simulink model "Disc"  (R2016b)
settings: Solver=VariableStepAuto  StartTime=0.0  StopTime=inf  RelTol=1e-3
undefined symbols (not defined in the file or in its folder): gray, Horn, Rec, Schunck, SDTV
libraries: visionstatistics x1, visionconversions x1, visiontextngfix x1, dspvision x1, visionanalysis x1
settings Model: Creator=shaurya  LastModifiedBy=Anushri-MacBook

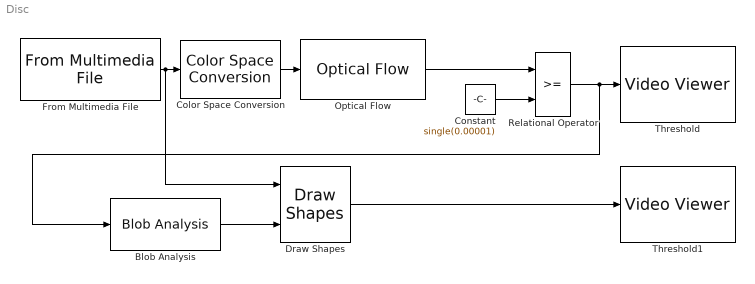
== system Disc ==
  " Threshold" : VideoViewer  colormapValue=gray(256)  FigPos=[617 607 476 443]  trueSizedOnce=on
  " Threshold1" : VideoViewer  colormapValue=gray(256)  FigPos=[140 607 476 443]  trueSizedOnce=on
  Blob Analysis : visionstatistics/Blob Analysis  Tag=vipblks_row_conv  area=off  centroid=off  bBox=on  majorAxis=off  minorAxis=off  angle=off  eccentricity=off  equivDiameterSq=off  extent=off  perimeter=off  maxBlobs=80  warnIfNumBlobsExceeded=on  isCount=off  useMinArea=on  minArea=200  useMaxArea=on  maxArea=400  excludeBorderBlob=on  outDT=double  isOutVarDim=on  isFill=on  fillValues=-1  conn=4  isLabel=off  outputMode=Binary point scaling  outputWordLength=32  outputFracLength=16  firstCoeffMode=Binary point scaling  firstCoeffWordLength=16  firstCoeffFracLength=14  secondCoeffMode=Binary point scaling  secondCoeffWordLength=32  secondCoeffFracLength=16  accumMode=Binary point scaling  accumWordLength=32  accumFracLength=0  prodOutputMode=Binary point scaling  prodOutputWordLength=32  prodOutputFracLength=16  roundingMode=Floor  overflowMode=off
  Color Space Conversion : visionconversions/Color Space  Conversion  conversion=Obsolete  conversionActive=R'G'B' to intensity  wp_str=D65  rec=Rec. 601 (SDTV)  sys=1125/60/2:1  imagePorts=One multidimensional signal
  Constant : Constant  Value=single(0.00001)
  Draw Shapes : visiontextngfix/Draw Shapes  shape=Rectangles  fill=off  lineWidth=1  fillClrSource=Specify via dialog  display=User-specified value  intensity=200  color=[0 1 0]  opacity=0.6  viewport=Entire image  antialiasing=off  inType=Obsolete  imagePorts=One multidimensional signal  prodOutputMode=Binary point scaling  prodOutputWordLength=32  prodOutputFracLength=14  memoryMode=Specify word length  memoryWordLength=16  memoryFracLength=15  roundingMode=Floor  overflowMode=off
  From Multimedia File : dspvision/From Multimedia File  inputFilename=/Users/Anushri-MacBook/Documents/MATLAB/final.mp4  loop=on  numPlays=inf  outputStreams=Video only  videoDataType=single  audioDataType=int16  inheritSampleTime=on  userDefinedSampleTime=1/30  noAudioOutput=off  isIntensityVideo=off  fourcc=RGB  colorVideoFormat=One multidimensional signal  outputEOF=off  dataOrg=Column-major  audioFrameSize=1024  computeAudioFrameSize=off  outSamplingMode=Sample based
  Optical Flow : visionanalysis/Optical Flow  method=Horn-Schunck  gradMethod=Difference filter [-1 1]  which2img=Current frame and N-th frame back  N=1  outVelForm=Magnitude-squared  lambda=1  stop_criteria=When maximum number of iterations is reached  maxAllowAbsDiff=eps  maxIter=1  numInports=3  sigmaS=1.5  sigmaW=1  eigTh=0.01  discardNormalFlow=off  outputCurrentImage=off  prodOutputMode=Binary point scaling  prodOutputWordLength=32  prodOutputFracLength=20  outputMode=Binary point scaling  outputWordLength=32  outputFracLength=20  roundingMode=Nearest  overflowMode=on
  Relational Operator : RelationalOperator  OutDataTypeStr=boolean  RndMeth=Nearest
  wires:
  From Multimedia File/1 -> Draw Shapes/1, Color Space Conversion/1
  Color Space Conversion/1 -> Optical Flow/1
  Optical Flow/1 -> Relational Operator/1
  Constant/1 -> Relational Operator/2
  Blob Analysis/1 -> Draw Shapes/2
  Draw Shapes/1 -> " Threshold1"/1
  Relational Operator/1 -> " Threshold"/1, Blob Analysis/1
